simulink model "quaternion2euler"  (Simulink 6.2)
settings: Solver=ode45  StartTime=0.0  StopTime=10.0  RelTol=1e-3
settings Model: Creator=krage  LastModifiedBy=Mads  ExtModeAutoUpdateStatusClock=off
settings OptimizationCC: InlineInvariantSignals=on
settings DebuggingCC: SolverPrmCheckMsg=warning

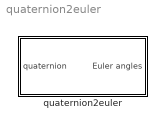
== system quaternion2euler ==
  quaternion2euler : Subsystem

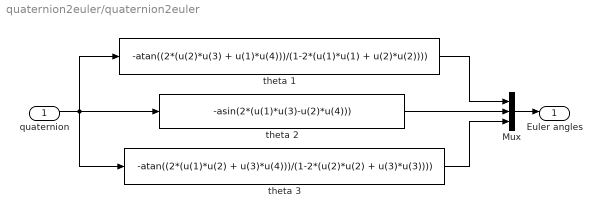
== system quaternion2euler/quaternion2euler ==
  quaternion : Inport  Port=1  LatchInput=off
  Mux : Mux  Inputs=3
  theta 1 : Fcn  Expr=-atan((2*(u(2)*u(3) + u(1)*u(4)))/(1-2*(u(1)*u(1) + u(2)*u(2))))
  theta 2 : Fcn  Expr=-asin(2*(u(1)*u(3)-u(2)*u(4)))
  theta 3 : Fcn  Expr=-atan((2*(u(1)*u(2) + u(3)*u(4)))/(1-2*(u(2)*u(2) + u(3)*u(3))))
  Euler angles : Outport
  wires:
  theta 1/1 -> Mux/1
  theta 2/1 -> Mux/2
  theta 3/1 -> Mux/3
  quaternion/1 -> theta 2/1, theta 1/1, theta 3/1
  Mux/1 -> Euler angles/1
